simulink model "Control System Implementation"  (R2015a)
settings: Solver=ode45  StartTime=0.0  StopTime=300  RelTol=1e-3
libraries: simulink x2
settings Model: Creator=Wen  LastModifiedBy=Wen

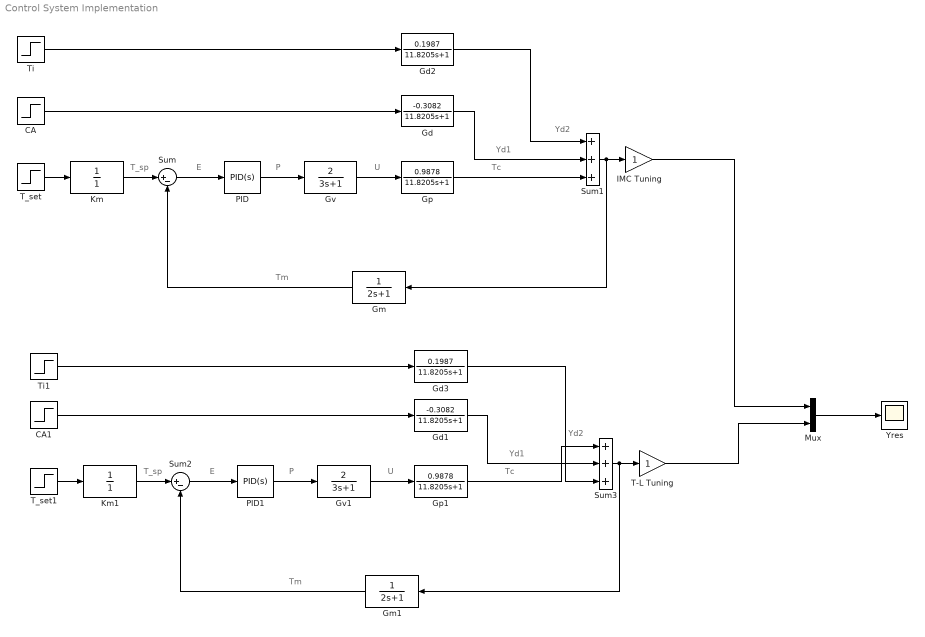
== system Control System Implementation ==
  note: Yd1
  note: Tc
  note: Yd2
  note: U
  note: P
  note: E
  note: T_sp
  note: Tm
  note: Yd1
  note: Tc
  note: Yd2
  note: U
  note: P
  note: E
  note: T_sp
  note: Tm
  " PID" : simulink/Continuous/PID Controller  Controller=PID  TimeDomain=Continuous-time  SampleTime=-1  IntegratorMethod=Forward Euler  FilterMethod=Forward Euler  Form=Ideal  UseFilter=on  ControllerParametersSource=internal  P=5.9832  I=1/11.8205  D=1  N=100  InitialConditionSource=internal  InitialConditionForIntegrator=0  InitialConditionForFilter=0  ExternalReset=none  LimitOutput=off  UpperSaturationLimit=inf  LowerSaturationLimit=-inf  LinearizeAsGain=on  AntiWindupMode=none  Kb=1  TrackingMode=off  Kt=1  PParamMin=[]  PParamMax=[]  IParamMin=[]  IParamMax=[]  DParamMin=[]  DParamMax=[]  NParamMin=[]  NParamMax=[]  KbParamMin=[]  KbParamMax=[]  KtParamMin=[]  KtParamMax=[]  POutMin=[]  POutMax=[]  IOutMin=[]  IOutMax=[]  DOutMin=[]  DOutMax=[]  NOutMin=[]  NOutMax=[]  KbOutMin=[]  KbOutMax=[]  KtOutMin=[]  KtOutMax=[]  IntegratorOutMin=[]  IntegratorOutMax=[]  FilterOutMin=[]  FilterOutMax=[]  SumOutMin=[]  SumOutMax=[]  SumI1OutMin=[]  SumI1OutMax=[]  SumI2OutMin=[]  SumI2OutMax=[]  SumI3OutMin=[]  SumI3OutMax=[]  SumDOutMin=[]  SumDOutMax=[]  SaturationOutMin=[]  SaturationOutMax=[]  IntegratorContinuousStateAttributes=''  IntegratorStateMustResolveToSignalObject=off  IntegratorRTWStateStorageClass=Auto  FilterContinuousStateAttributes=''  FilterStateMustResolveToSignalObject=off  FilterRTWStateStorageClass=Auto  DifferentiatorICPrevScaledInput=0  DifferentiatorOutMin=[]  DifferentiatorOutMax=[]
  " PID1" : simulink/Continuous/PID Controller  Controller=PID  TimeDomain=Continuous-time  SampleTime=-1  IntegratorMethod=Forward Euler  FilterMethod=Forward Euler  Form=Ideal  UseFilter=on  ControllerParametersSource=internal  P=3.2143  I=1/28.3840  D=2/0479  N=100  InitialConditionSource=internal  InitialConditionForIntegrator=0  InitialConditionForFilter=0  ExternalReset=none  LimitOutput=off  UpperSaturationLimit=inf  LowerSaturationLimit=-inf  LinearizeAsGain=on  AntiWindupMode=none  Kb=1  TrackingMode=off  Kt=1  PParamMin=[]  PParamMax=[]  IParamMin=[]  IParamMax=[]  DParamMin=[]  DParamMax=[]  NParamMin=[]  NParamMax=[]  KbParamMin=[]  KbParamMax=[]  KtParamMin=[]  KtParamMax=[]  POutMin=[]  POutMax=[]  IOutMin=[]  IOutMax=[]  DOutMin=[]  DOutMax=[]  NOutMin=[]  NOutMax=[]  KbOutMin=[]  KbOutMax=[]  KtOutMin=[]  KtOutMax=[]  IntegratorOutMin=[]  IntegratorOutMax=[]  FilterOutMin=[]  FilterOutMax=[]  SumOutMin=[]  SumOutMax=[]  SumI1OutMin=[]  SumI1OutMax=[]  SumI2OutMin=[]  SumI2OutMax=[]  SumI3OutMin=[]  SumI3OutMax=[]  SumDOutMin=[]  SumDOutMax=[]  SaturationOutMin=[]  SaturationOutMax=[]  IntegratorContinuousStateAttributes=''  IntegratorStateMustResolveToSignalObject=off  IntegratorRTWStateStorageClass=Auto  FilterContinuousStateAttributes=''  FilterStateMustResolveToSignalObject=off  FilterRTWStateStorageClass=Auto  DifferentiatorICPrevScaledInput=0  DifferentiatorOutMin=[]  DifferentiatorOutMax=[]
  CA : Step  Time=20  After=-50  SampleTime=0
  CA1 : Step  Time=20  After=-50  SampleTime=0
  Gd : TransferFcn  Numerator=[-0.3082]  Denominator=[11.8205 1]
  Gd1 : TransferFcn  Numerator=[-0.3082]  Denominator=[11.8205 1]
  Gd2 : TransferFcn  Numerator=[0.1987]  Denominator=[11.8205 1]
  Gd3 : TransferFcn  Numerator=[0.1987]  Denominator=[11.8205 1]
  Gm : TransferFcn  Denominator=[2 1]
  Gm1 : TransferFcn  Denominator=[2 1]
  Gp : TransferFcn  Numerator=[0.9878]  Denominator=[11.8205 1]
  Gp1 : TransferFcn  Numerator=[0.9878]  Denominator=[11.8205 1]
  Gv : TransferFcn  Numerator=[2]  Denominator=[3 1]
  Gv1 : TransferFcn  Numerator=[2]  Denominator=[3 1]
  IMC Tuning : Gain
  Km : TransferFcn  Denominator=[1]
  Km1 : TransferFcn  Denominator=[1]
  Mux : Mux  Inputs=2
  Sum : Sum  Inputs=|+-
  Sum1 : Sum  Inputs=+++
  Sum2 : Sum  Inputs=|+-
  Sum3 : Sum  Inputs=+++
  T-L Tuning : Gain
  T_set : Step  Time=200  After=5  SampleTime=0
  T_set1 : Step  Time=200  After=5  SampleTime=0
  Ti : Step  Time=100  After=20  SampleTime=0
  Ti1 : Step  Time=100  After=20  SampleTime=0
  Yres : Scope
      settings: ShowLegends=on  YMin=-0.1  YMax=0.3
  wires:
  Sum/1 -> " PID"/1
  " PID"/1 -> Gv/1
  Sum1/1 -> Gm/1, IMC Tuning/1
  T_set/1 -> Km/1
  Gv/1 -> Gp/1
  Gm/1 -> Sum/2
  Km/1 -> Sum/1
  Gp/1 -> Sum1/3
  IMC Tuning/1 -> Mux/1
  Gd/1 -> Sum1/2
  CA/1 -> Gd/1
  Ti/1 -> Gd2/1
  Gd2/1 -> Sum1/1
  Sum2/1 -> " PID1"/1
  " PID1"/1 -> Gv1/1
  Sum3/1 -> Gm1/1, T-L Tuning/1
  T_set1/1 -> Km1/1
  Gv1/1 -> Gp1/1
  Gm1/1 -> Sum2/2
  Km1/1 -> Sum2/1
  Gp1/1 -> Sum3/1
  T-L Tuning/1 -> Mux/2
  Gd1/1 -> Sum3/2
  CA1/1 -> Gd1/1
  Ti1/1 -> Gd3/1
  Gd3/1 -> Sum3/3
  Mux/1 -> Yres/1
